simulink model "Basic_Parachute_Dynamics_Simulink_Model"  (R2017b)
settings: Solver=ode23  StartTime=0.0  StopTime=250  MaxStep=0.01  RelTol=1e-3  AbsTol=1E-6  EnableMultiTasking=on
values from neighbouring files (symbols this model uses):
  A_v = (pi/4)*D_v^2    (= 19.6349540849)    [Simple_Parachute_Sim_Constants.m]
  Cd_p = 0.95    [Simple_Parachute_Sim_Constants.m]
  Cd_v = 1.3    [Simple_Parachute_Sim_Constants.m]
  D_p = 35.36    [Simple_Parachute_Sim_Constants.m]
  g = -9.80665    [Simple_Parachute_Sim_Constants.m]
  M_p = 113.4    [Simple_Parachute_Sim_Constants.m]
  M_v = 10829.52    [Simple_Parachute_Sim_Constants.m]
  N = 3    [Simple_Parachute_Sim_Constants.m]
  V0 = -58    [Simple_Parachute_Sim_Constants.m]
  X0 = 2750    [Simple_Parachute_Sim_Constants.m]
  x1 = 3.979E-09    (= 3.979e-09)    [Simple_Parachute_Sim_Constants.m]
  x2 = -0.000117    [Simple_Parachute_Sim_Constants.m]
  x3 = 1.224    [Simple_Parachute_Sim_Constants.m]
  Z = Z*Z_Factor    [Simple_Parachute_Sim_Constants.m]
libraries: simulink x1
settings Model: Creator=The MathWorks, Inc.  LastModifiedBy=Pele
settings SolverCC: ZeroCrossAlgorithm=Adaptive
settings DataIOCC: MaxDataPoints=7500  SaveFormat=Array  SaveOutput=off  SignalLogging=off  DSMLogging=off  SaveTime=off
settings OptimizationCC: ExpressionDepthLimit=2147483647  EfficientFloat2IntCast=on  LifeSpan=inf
settings DebuggingCC: UnderspecifiedInitializationDetection=Classic  MergeDetectMultiDrivingBlocksExec=none  IgnoredZcDiagnostic=none  FcnCallInpInsideContextMsg=warning  StateNameClashWarn=warning  SFUnexpectedBacktrackingDiag=warning  SFNoUnconditionalDefaultTransitionDiag=warning  SFExecutionAtInitializationDiag=none
settings HardwareCC: ProdBitPerPointer=32  ProdBitPerSizeT=32  ProdBitPerPtrDiffT=32  ProdLargestAtomicFloat=None  ProdIntDivRoundTo=Undefined  ProdEndianess=Unspecified  ProdWordSize=32  ProdHWDeviceType=32-bit Generic  TargetBitPerPointer=64  TargetBitPerSizeT=64  TargetBitPerPtrDiffT=64  TargetLongLongMode=on  TargetIntDivRoundTo=Zero  TargetEndianess=LittleEndian  TargetWordSize=64  TargetHWDeviceType=MATLAB Host  ProdEqTarget=off
settings ModelReferenceCC: PropagateSignalLabelsOutOfModel=off
settings RTWCC: SystemTargetFile=rsim.tlc  TemplateMakefile=rsim_default_tmf  Description=Rapid Simulation Target
settings CodeAppCC: StateflowObjectComments=on
settings TargetCC: ParMdlRefBuildCompliant=on  ConcurrentExecutionCompliant=on  MatFileLogging=on
settings ConfigComp: CovMetricSettings=dw  CovHtmlReporting=on  CovSaveCumulativeToWorkspaceVar=on  CovSaveSingleToWorkspaceVar=on  CovExternalEMLEnable=off

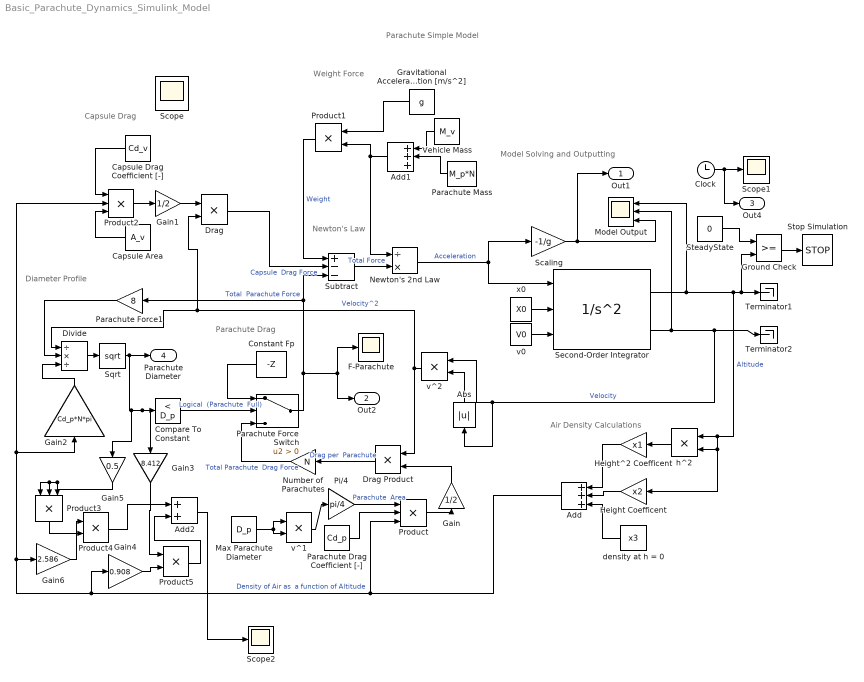
== system Basic_Parachute_Dynamics_Simulink_Model ==
  note: Diameter Profile
  note: Model Solving and Outputting
  note: Newton's Law
  note: Weight Force
  note: Capsule Drag
  note: Parachute Drag
  note: Air Density Calculations
  note: Parachute Simple Model
  Abs : Abs
  Add : Sum  Inputs=+++
  Add1 : Sum  Inputs=+++
  Add2 : Sum
  "Capsule Area " : Constant  Value=A_v
  Capsule Drag Coefficient [-] : Constant  Value=Cd_v
  Clock : Clock
  Compare To Constant : simulink/Logic and Bit Operations/Compare To Constant  relop=<  const=D_p  OutDataTypeStr=boolean
  Constant Fp : Constant  Value=-Z
  Divide : Product  Inputs=/*/
  "Drag " : Product
  Drag Product : Product
  F-Parachute : Scope
  Gain : Gain  Gain=1/2
  Gain1 : Gain  Gain=1/2
  Gain2 : Gain  Gain=Cd_p*N*pi
  Gain3 : Gain  Gain=8.412
  Gain4 : Gain  Gain=0.908
  Gain5 : Gain  Gain=0.5
  Gain6 : Gain  Gain=2.586
  Gravitational Acceleration [m/s^2] : Constant  Value=g
  Ground Check : RelationalOperator  OutDataTypeStr=boolean  RndMeth=Simplest
  Height Coefficent : Gain  Gain=x2
  Height^2 Coefficent : Gain  Gain=x1
  Max Parachute Diameter : Constant  Value=D_p
  Model Output : Scope  NumInputPorts=3
  Newton's 2nd Law : Product  Inputs=/*
  "Number of Parachutes " : Gain  Gain=N
  "Parachute Force Switch  " : Switch  Criteria=u2 > Threshold
  Parachute Mass : Constant  Value=M_p*N
  Parachute Drag Coefficient [-] : Constant  Value=Cd_p
  Parachute Force1 : Gain  Gain=8
  Pi/4 : Gain  Gain=pi/4
  Product : Product  Inputs=3
  Product1 : Product
  Product2 : Product  Inputs=3
  Product3 : Product  Inputs=3
  Product4 : Product
  Product5 : Product
  Scaling : Gain  Gain=-1/g
  Scope1 : Scope
  Scope2 : Scope
  Second-Order Integrator : SecondOrderIntegrator  ICSourceX=external  ICX=20  LimitX=on  LowerLimitX=0.0  StateNameX='Position'  ICSourceDXDT=external  StateNameDXDT='Velocity'
  Sqrt : Sqrt  SaturateOnIntegerOverflow=on
  SteadyState : Constant  Value=0
  Stop Simulation : Stop
  Subtract : Sum  Inputs=+--
  Terminator1 : Terminator
  Terminator2 : Terminator
  Vehicle Mass : Constant  Value=M_v
  density at h = 0 : Constant  Value=x3
  h^2 : Product
  "v0 " : Constant  Value=V0
  v^1 : Product
  v^2 : Product
  x0 : Constant  Value=X0
  Out1 : Outport
  Out2 : Outport  Port=2
  Out4 : Outport  Port=3
  Parachute Diameter : Outport  Port=4
  Scope : Scope
  wires:
  Second-Order Integrator/1 -> Model Output/1, Ground Check/2, Terminator1/1, h^2/1, Height Coefficent/1, h^2/2  "Altitude"
  Second-Order Integrator/2 -> Model Output/2, v^2/1, Abs/1, Terminator2/1  "Velocity"
  x0/1 -> Second-Order Integrator/2
  Product/1 -> Gain/1
  Gain/1 -> Drag Product/2
  v^2/1 -> Drag Product/1, "Drag "/2, Divide/1  "Velocity^2"
  Drag Product/1 -> "Number of Parachutes "/1  "Drag per  Parachute"
  Newton's 2nd Law/1 -> Scaling/1, Second-Order Integrator/1  "Acceleration"
  Pi/4/1 -> Product/1  "Parachute  Area"
  Abs/1 -> v^2/2
  "v0 "/1 -> Second-Order Integrator/3
  h^2/1 -> Height^2 Coefficent/1
  Height^2 Coefficent/1 -> Add/1
  Height Coefficent/1 -> Add/2
  density at h = 0/1 -> Add/3
  Add/1 -> Gain4/1, Gain2/1, Product2/2, Gain6/1, Product/3  "Density of Air as  a function of Altitude"
  Subtract/1 -> Newton's 2nd Law/2  "Total Force"
  Product2/1 -> Gain1/1
  Product1/1 -> Subtract/1  "Weight"
  Capsule Drag Coefficient [-]/1 -> Product2/1
  Gain1/1 -> "Drag "/1
  "Number of Parachutes "/1 -> "Parachute Force Switch  "/3  "Total Parachute  Drag Force"
  "Drag "/1 -> Subtract/2  "Capsule  Drag Force"
  Ground Check/1 -> Stop Simulation/1
  Scaling/1 -> Out1/1, Model Output/3
  Clock/1 -> Out4/1, Scope1/1
  Gravitational Acceleration [m/s^2]/1 -> Product1/1
  SteadyState/1 -> Ground Check/1
  "Capsule Area "/1 -> Product2/3
  "Parachute Force Switch  "/1 -> Subtract/3, Parachute Force1/1, Out2/1, F-Parachute/1  "Total  Parachute Force"
  Gain2/1 -> Divide/3
  Parachute Force1/1 -> Divide/2
  Divide/1 -> Sqrt/1
  Sqrt/1 -> Parachute Diameter/1, Gain5/1, Compare To Constant/1, Gain3/1
  Compare To Constant/1 -> "Parachute Force Switch  "/2  "Logical  (Parachute  Full)"
  Constant Fp/1 -> "Parachute Force Switch  "/1
  Parachute Drag Coefficient [-]/1 -> Product/2
  Max Parachute Diameter/1 -> v^1/2, v^1/1
  v^1/1 -> Pi/4/1
  Vehicle Mass/1 -> Add1/1
  Add1/1 -> Product1/2, Newton's 2nd Law/1
  Gain5/1 -> Product3/1, Product3/2, Product3/3
  Gain6/1 -> Product4/1
  Product3/1 -> Product4/2
  Gain4/1 -> Product5/2
  Gain3/1 -> Product5/1
  Product5/1 -> Add2/2
  Product4/1 -> Add2/1
  Add2/1 -> Scope2/1
  Parachute Mass/1 -> Add1/2
